simulink library "SimulatorLibrary"  (R2016a)
settings: Solver=VariableStepAuto  StartTime=0.0  StopTime=10.0  RelTol=1e-3
settings Model: Creator=MortenFyhn  LastModifiedBy=vegard
settings DataIOCC: LimitDataPoints=on
settings DebuggingCC: AllowSymbolicDim=off
settings ModelReferenceCC: PropagateSignalLabelsOutOfModel=off
settings GRTTargetCC: GeneratePreprocessorConditionals=Use local settings

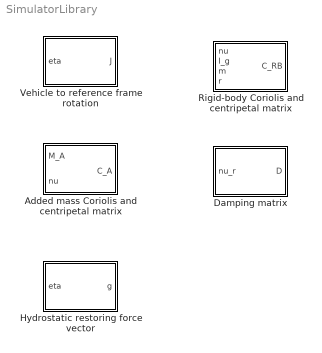
== system SimulatorLibrary ==
  Added mass Coriolis and centripetal matrix : MATLAB Function  TreatAsAtomicUnit=on
  Damping matrix : MATLAB Function  TreatAsAtomicUnit=on
  Hydrostatic restoring force vector : MATLAB Function  TreatAsAtomicUnit=on
  Rigid-body Coriolis and centripetal matrix : MATLAB Function  TreatAsAtomicUnit=on
  Vehicle to reference frame rotation : MATLAB Function  TreatAsAtomicUnit=on

== matlab function SimulatorLibrary/Vehicle to reference frame rotation ==
  data: eta input; J output
function J = fcn(eta)
%#codegen
phi = eta(4);
theta = eta(5);
psi = eta(6);

R = Reuler([phi theta psi]');
T = [1 sin(phi)*tan(theta) cos(phi)*tan(theta)
     0            cos(phi)           -sin(phi)
     0 sin(phi)/cos(theta) cos(phi)/cos(theta)];

J = [   R     zeros(3)
     zeros(3)    T    ];

== matlab function SimulatorLibrary/Added mass Coriolis and centripetal matrix ==
  data: M_A input; nu input; C_A output
function C_A = fcn(M_A, nu)
%#codegen

v = nu(1:3);
omega = nu(4:6);
A_11 = M_A(1:3,1:3);
A_12 = M_A(1:3,4:6);
A_21 = M_A(4:6,1:3);
A_22 = M_A(4:6,4:6);

C_A_11 = zeros(3);
C_A_12 = -skew(A_11*v + A_12*omega);
C_A_21 = C_A_12;
C_A_22 = -skew(A_21*v + A_22*omega);

C_A = [C_A_11 C_A_12;
       C_A_21 C_A_22];

== matlab function SimulatorLibrary/Rigid-body Coriolis and centripetal matrix ==
  data: nu input; I_g input; m input; C_RB output; r input
function C_RB = fcn(nu, I_g, m, r)
%#codegen

omega = nu(4:6);

C_RB_CG = [m*skew(omega)         zeros(3)
                zeros(3) -skew(I_g*omega)];
            
H = Hmatrix(r);

C_RB = H' * C_RB_CG * H;

== matlab function SimulatorLibrary/Damping matrix ==
  data: nu_r input; D output
function D = fcn(nu_r)
%#codegen

% from (2.36), (2.37), (2.38) p. 25 in PhD
% D_linear and D_n are determined from experiments

% D_linear is the linear damping matrix
% D > 0, must have positive damping
X_u = -1;
Y_v = -1;
Z_w = -1;
K_p = -1;
M_q = -1;
N_r = -1;

x = [X_u, Y_v, Z_w, K_p, M_q, N_r];
D_linear = -diag(x);

% D_n is the quadratic damping, 
% mostly caused by vortex shedding
X_uu = -1;
Y_vv = -1;
Z_ww = -1;
K_pp = -1;
M_qq = -1;
N_rr = -1;

y = [X_uu*abs(nu_r(1)), 
    Y_vv*abs(nu_r(2)),
    Z_ww*abs(nu_r(3)),
    K_pp*abs(nu_r(4)),
    M_qq*abs(nu_r(5)),
    N_rr*abs(nu_r(6))]
D_n = -diag(y);

% alpha is a tuning parameter
alpha = 1;
D = D_linear*exp(-alpha*norm(nu_r)) + D_n;

== matlab function SimulatorLibrary/Hydrostatic restoring force vector ==
  data: eta input; g output
function g = fcn(eta) %#ok<INUSD>
%#codegen

g = zeros(6,1);
